simulink model "CryoDetFP"  (R2015b)
settings: Solver=ode45  SolverMode=SingleTasking  StartTime=0.0  StopTime=10e-5  MaxStep=1e-9  RelTol=1e-3
values from neighbouring files (symbols this model uses):
  Fclk = Fadc/2    (= 185000000)    [setupCryoFPGA.m]    (also in setupCryoNew.m)
  freqBusAddrBits = 4    [setupCryoNew.m]
  noise = ifft(exp(2i*pi*rand(1, noiseLen)) .* fft(fir1(noiseLen-1, noiseBW/Fclk*noiseSteps)))    [setupCryoFPGA.m]    (also in setupCryoNew.m = exp(2i*pi*rand(1, noiseLen)))
  noiseLen = 128    [setupCryoFPGA.m]    (also in setupCryoNew.m)
  noiseSteps = 32    [setupCryoFPGA.m]    (also in setupCryoNew.m)
  notch = tf( [1 a*wNotch/Q wNotch^2], [1 wNotch/Q wNotch^2])    [setupCryoNew.m]
  notch2 = tf( [1 a*wNotch/Q wNotch^2], [1 wNotch/Q wNotch^2])    [setupCryoNew.m]
  Tclk = 1/Fclk    (= 5.40540540541e-09)    [setupCryoFPGA.m]    (also in setupCryoNew.m)
undefined symbols (not defined in the file or in its folder): AXI4, Lite, notch3, notch4, xlipgetpartsetting
libraries: xbsIndex_r4 x1085
(part 2 of 8)

== system CryoDetFP/DspCore/AdcDac 0/Ref Delay ==
  note: Delays DAC output data used as Reference for input signal
      | Delay is to compensate for delay of DAC (big), up/downconverter, cable plant, cryostat etc.
      | This is to prevent too much delay mismatch from winding up phase vs. frequency of S21's of sidebands wrt to central line
  In1 : Inport
  Addressable Shift Register : xbsIndex_r4/Addressable Shift Register  infer_latency=on  depth=2  initVector=[0]  en=off  use_behavioral_HDL=on  Optimization=Resource  dbl_ovrd=off  block_type=addrsr
      settings: infoedit="Delay of configurable length.  Any element in the delay line can be addressed and driven onto the output port.<br><br>Hardware notes: Generates fast, compact FIFO-style shift registers or delay lines using SRL16/SRL32 mode of the slice LUTs"
  Addressable Shift Register1 : xbsIndex_r4/Addressable Shift Register  infer_latency=on  depth=2  initVector=[0]  en=off  use_behavioral_HDL=on  Optimization=Resource  dbl_ovrd=off  block_type=addrsr
      settings: infoedit="Delay of configurable length.  Any element in the delay line can be addressed and driven onto the output port.<br><br>Hardware notes: Generates fast, compact FIFO-style shift registers or delay lines using SRL16/SRL32 mode of the slice LUTs"
  Demux : Demux  Outputs=2
  Display : Display
      settings: Decimation=128
  Gateway Out : xbsIndex_r4/Gateway Out  inherit_from_input=off  hdl_port=off  rows=1  columns=1  UseAsDAC=off  DACChannel='1'  interface=None  automatic_assignment=on  address_offset=hex2dec('00')  intf_name=''  intf_description=''  timing_constraint=None  locs_specified=off  LOCs={}  io_standard={}  block_type=gatewayout
  Mux : Mux  Inputs=2
  Out1 : Outport
  wires:
  Addressable Shift Register/1 -> Mux/1
  Addressable Shift Register1/1 -> Mux/2
  In1/1 -> Demux/1
  Demux/2 -> Addressable Shift Register1/1
  Demux/1 -> Addressable Shift Register/1
  [refDel] -> Addressable Shift Register1/2, Addressable Shift Register/2, Gateway Out/1
  Mux/1 -> Out1/1
  Gateway Out/1 -> Display/1

== system CryoDetFP/DspCore/AdcDac 0/SBmodulator ==
  note: To DAC
  note: From tone generators
  note: to sideband demodulators
  note: Band-limited white noise
      | modulator
  note: AM generator
  note: Sideband Modulator
      | Produce sidebands at offset frequency specified by dFsb via amplitude modulation
      | Ampl1 is ratio of sidebands to central line, must be <<1
      | Also provides enable/disable for RF
      | and whitenoise modulator
  In1 : Inport
  AddSub : xbsIndex_r4/AddSub  mode=Addition  use_carryin=off  use_carryout=off  en=off  latency=1  precision=User Defined  arith_type="Signed  (2's comp)"  n_bits=16  bin_pt=15  quantization=Truncate  overflow=Wrap  use_behavioral_HDL=off  hw_selection=Fabric  pipelined=off  dbl_ovrd=off  block_type=addsub
  AddSub1 : xbsIndex_r4/AddSub  mode=Subtraction  use_carryin=off  use_carryout=off  en=off  latency=1  precision=User Defined  arith_type="Signed  (2's comp)"  n_bits=16  bin_pt=15  quantization=Truncate  overflow=Wrap  use_behavioral_HDL=off  hw_selection=Fabric  pipelined=off  dbl_ovrd=off  block_type=addsub
  Concat1 : xbsIndex_r4/Concat  num_inputs=2  dbl_ovrd=off  block_type=concat
  Constant : xbsIndex_r4/Constant  const=1.0  gui_display_data_type=Boolean  arith_type=Boolean  n_bits=16  bin_pt=14  preci_type=Single  exp_width=8  frac_width=24  explicit_period=off  period=1  equ=P=C  opselect=C  inp2=PCIN>>17  opr=+  inp1=P  carry=CIN  dbl_ovrd=off  block_type=constant
  Constant1 : xbsIndex_r4/Constant  const=1.0  gui_display_data_type=Fixed-point  arith_type=Signed (2's comp)  n_bits=16  bin_pt=15  preci_type=Single  exp_width=8  frac_width=24  explicit_period=off  period=1  equ=P=C  opselect=C  inp2=PCIN>>17  opr=+  inp1=P  carry=CIN  dbl_ovrd=off  block_type=constant
  Constant2 : xbsIndex_r4/Constant  const=0  gui_display_data_type=Fixed-point  arith_type=Signed (2's comp)  n_bits=16  bin_pt=15  preci_type=Single  exp_width=8  frac_width=24  explicit_period=off  period=1  equ=P=C  opselect=C  inp2=PCIN>>17  opr=+  inp1=P  carry=CIN  dbl_ovrd=off  block_type=constant
  Counter : xbsIndex_r4/Counter  cnt_type=Free Running  cnt_to=Inf  operation=Up  start_count=0  cnt_by_val=1  arith_type=Unsigned  n_bits=ceil(log2(noiseLen))  bin_pt=0  load_pin=off  rst=off  en=off  explicit_period=on  period=Tclk*noiseSteps  use_behavioral_HDL=off  implementation=Fabric  dbl_ovrd=off  block_type=counter
  "DDS Compiler 6.0 " : xbsIndex_r4/DDS Compiler 6.0   partspresent=Phase_Generator_and_SIN_COS_LUT  dds_clock_rate=Fclk/1e6  channels=1  mode_of_operation=Standard  modulus=9  parameter_entry=Hardware_Parameters  spurious_free_dynamic_range=45  frequency_resolution=0.4  noise_shaping=None  phase_width=16  output_width=16  output_selection=Sine_and_Cosine  negative_sine=off  negative_cosine=off  amplitude_mode=Unit_Circle  memory_type=Auto  optimization_goal=Speed  dsp48_use=Maximal  resync=off  latency_configuration=Auto  latency=5  has_phase_out=off  has_aclken=off  has_aresetn=off  explicit_period=on  period=Tclk  data_has_tlast=Not_Required  has_tready=off  s_phase_has_tuser=Not_Required  m_data_has_tuser=Not_Required  m_phase_has_tuser=Not_Required  s_phase_tuser_width=1  output_form=Twos_Complement  s_config_sync_mode=On_Vector  phase_increment=Programmable  output_frequency1=0  output_frequency2=0  output_frequency3=0  output_frequency4=0  output_frequency5=0  output_frequency6=0  output_frequency7=0  output_frequency8=0  output_frequency9=0  output_frequency10=0  output_frequency11=0  output_frequency12=0  output_frequency13=0  output_frequency14=0  output_frequency15=0  output_frequency16=0  pinc1='0'  pinc2='0'  pinc3='0'  pinc4='0'  pinc5='0'  pinc6='0'  pinc7='0'  pinc8='0'  pinc9='0'  pinc10='0'  pinc11='0'  pinc12='0'  pinc13='0'  pinc14='0'  pinc15='0'  pinc16='0'  phase_offset=None  phase_offset_angles1=0  phase_offset_angles2=0  phase_offset_angles3=0  phase_offset_angles4=0  phase_offset_angles5=0  phase_offset_angles6=0  phase_offset_angles7=0  phase_offset_angles8=0  phase_offset_angles9=0  phase_offset_angles10=0  phase_offset_angles11=0  phase_offset_angles12=0  phase_offset_angles13=0  phase_offset_angles14=0  phase_offset_angles15=0  phase_offset_angles16=0  poff1='0'  poff2='0'  poff3='0'  poff4='0'  poff5='0'  poff6='0'  poff7='0'  poff8='0'  poff9='0'  poff10='0'  poff11='0'  poff12='0'  poff13='0'  poff14='0'  poff15='0'  poff16='0'  trim_axipin_name=on  simulation_type=hybrid_sim  simulation_model=sysgen:xddsv6_0_cmodel  data_path_portlist={ 's_axis_config_tdata_poff', 's_axis_config_tdata_chan0_poff', 's_axis_config_tdata_pinc', 's_axis_config_tdata_chan0_pinc', 's_axis_phase_tdata_resync', 's_axis_phase_tdata_chan0_resync', 's_axis_phase_tdata_poff', 's_axis_phase_tdata_chan0_poff', 's_axis_phase_tdata_pinc', 's_axis_phase_tdata_chan0_pinc', 's_axis_phase_tdata_phase_in', 'm_axis_data_tdata_sine', 'm_axis_data_tdata_chan0_sine', 'm_axis_data_tdata_cosine', 'm_axis_data_tdata_chan0_cosine', 'm_axis_phase_tdata_phase_out', 'm_axis_phase_tdata_chan0_phase_out'}  por_mode=false  gui_behaviour=Sysgen  ip_name=DDS Compiler  ip_version=6.0  dsptool_ready=true  wrapper_available=true  port_translation_map={ 'aclken' => 'en', 'aresetn' => 'rst' }  ipcore_usecache=true  ipcore_useipmodelcache=true  ipcore_xco_need_fpga_part=true  ipcore_fpga_part=xlipgetpartsetting(gcb, {'kintex7', 'xc7k325t', '-3', 'fbg676'})  ipcore_verbose=false  block_type=dds_compiler_v6_0
  Demux : Demux  Outputs=2
  Gateway Out{,1..7} (8 alike) : xbsIndex_r4/Gateway Out  inherit_from_input=off  hdl_port=off  rows=1  columns=1  UseAsDAC=off  DACChannel='1'  interface=None  automatic_assignment=on  address_offset=hex2dec('00')  intf_name=''  intf_description=''  timing_constraint=None  locs_specified=off  LOCs={}  io_standard={}  block_type=gatewayout
  Modulator Control : Display
  Mult : xbsIndex_r4/Mult  precision=User Defined  arith_type="Signed  (2's comp)"  n_bits=16  bin_pt=15  quantization=Truncate  overflow=Wrap  en=off  latency=3  use_behavioral_HDL=off  opt=Speed  use_embedded=on  optimum_pipeline=off  pipeline=on  dbl_ovrd=off  use_rpm=on  placement_style=Triangular  block_type=mult
  Mult1 : xbsIndex_r4/Mult  precision=User Defined  arith_type="Signed  (2's comp)"  n_bits=16  bin_pt=15  quantization=Truncate  overflow=Wrap  en=off  latency=3  use_behavioral_HDL=off  opt=Speed  use_embedded=on  optimum_pipeline=off  pipeline=on  dbl_ovrd=off  use_rpm=on  placement_style=Triangular  block_type=mult
  Mult2 : xbsIndex_r4/Mult  precision=User Defined  arith_type="Signed  (2's comp)"  n_bits=16  bin_pt=15  quantization=Truncate  overflow=Wrap  en=off  latency=3  use_behavioral_HDL=off  opt=Speed  use_embedded=on  optimum_pipeline=off  pipeline=on  dbl_ovrd=off  use_rpm=on  placement_style=Triangular  block_type=mult
  Mux : Mux  Inputs=2
  Mux1 : xbsIndex_r4/Mux  inputs=4  en=off  latency=1  precision=User Defined  arith_type="Signed  (2's comp)"  n_bits=16  bin_pt=15  quantization=Truncate  overflow=Flag as error  dbl_ovrd=off  block_type=mux
  Mux2 : xbsIndex_r4/Mux  inputs=4  en=off  latency=1  precision=User Defined  arith_type="Signed  (2's comp)"  n_bits=16  bin_pt=15  quantization=Truncate  overflow=Flag as error  dbl_ovrd=off  block_type=mux
  Phase Modulator : Subsystem
  ROM : xbsIndex_r4/ROM  depth=noiseLen  initVector=real(noise)  distributed_mem=Block RAM  rst=off  init_reg=0  en=off  latency=1  gui_display_data_type=Fixed-point  arith_type="Signed  (2's comp)"  n_bits=16  bin_pt=15  preci_type=Single  exp_width=8  frac_width=24  optimize=Area  use_rpm=on  dbl_ovrd=off  block_type=sprom
  ROM1 : xbsIndex_r4/ROM  depth=noiseLen  initVector=imag(noise)  distributed_mem=Block RAM  rst=off  init_reg=0  en=off  latency=1  gui_display_data_type=Fixed-point  arith_type="Signed  (2's comp)"  n_bits=16  bin_pt=15  preci_type=Single  exp_width=8  frac_width=24  optimize=Area  use_rpm=on  dbl_ovrd=off  block_type=sprom
  Scope : Scope  NumInputPorts=4
  Terminator : Terminator
  sideband LO : Scope  NumInputPorts=3
  Out1 : Outport
  tag scope: SBI=global, SBQ=global
  wires:
  [dFsb] -> "DDS Compiler 6.0 "/2
  Constant/1 -> "DDS Compiler 6.0 "/1
  Mult/1 -> AddSub/1
  Constant1/1 -> AddSub1/1
  [Ampl1] -> AddSub1/2, Mult/2
  AddSub1/1 -> AddSub/2
  "DDS Compiler 6.0 "/1 -> Terminator/1
  Counter/1 -> ROM1/1, ROM/1
  Demux/1 -> Mult2/1, Phase Modulator/1(Iin)
  Demux/2 -> Phase Modulator/2(Qin), Mult1/1
  Gateway Out/1 -> Scope/1
  Gateway Out1/1 -> Scope/2
  Gateway Out2/1 -> Scope/3
  Gateway Out3/1 -> Scope/4
  "DDS Compiler 6.0 "/3 -> Gateway Out4/1, [SBI], Mult/1
  "DDS Compiler 6.0 "/2 -> Gateway Out5/1, [SBQ]
  Gateway Out4/1 -> sideband LO/1
  Gateway Out5/1 -> sideband LO/2
  [RFen] -> Concat1/2
  Concat1/1 -> Gateway Out6/1, Mux1/1, Mux2/1
  [whiteNoiseGen] -> Concat1/1
  AddSub/1 -> Gateway Out7/1, Mult1/2, Mult2/2
  ROM/1 -> Gateway Out2/1, Phase Modulator/3(Ipm)
  ROM1/1 -> Gateway Out3/1, Phase Modulator/4(Qpm)
  Constant2/1 -> Mux2/4, Mux1/2, Mux1/4, Mux2/2
  Mux2/1 -> Mux/1, Gateway Out/1
  Mux1/1 -> Mux/2, Gateway Out1/1
  Phase Modulator/1(Iout) -> Mux2/5
  Phase Modulator/2(Qout) -> Mux1/5
  Mult2/1 -> Mux2/3
  Mult1/1 -> Mux1/3
  Gateway Out6/1 -> Modulator Control/1
  Gateway Out7/1 -> sideband LO/3
  In1/1 -> Demux/1
  Mux/1 -> Out1/1

== system CryoDetFP/DspCore/AdcDac 0/dF ==
  note: eta Ram has latency 2
  note: sig0
  note: conj(Ref0)
  note: Match latencies
  note: dF
  note: Ref
  note: Sig
  note: Frequency error dF = Im(eta'*Ref'*Sig)
      | where eta' is like a phase and amplitude calibration including the phase determined by the 2 sidebands and amplitude determined by the reference central line and bandwidth
      |
      | get channel ID
      | fetch eta'
      | calc dF
  note: Bandwidth (kludge in with constant for now)
  In1 : Inport
  etaBus : Inport  Port=2
  Bus Creator : BusCreator  Inputs=2
  Bus Selector : BusSelector  OutputSignals=chanAndTvalid,signal2
  CMult : xbsIndex_r4/CMult  const=-1  gui_display_data_type=Floating-point  const_n_bits=24  const_bin_pt=22  float_type=Single  exp_bits=8  fraction_bits=24  en=off  latency=1  precision=Full  arith_type="Signed  (2's comp)"  n_bits=24  bin_pt=22  quantization=Truncate  overflow=Wrap  use_behavioral_HDL=on  mem_type=Distributed RAM  pipeline=off  dbl_ovrd=off  block_type=cmult
  Constant : xbsIndex_r4/Constant  const=0  gui_display_data_type=Fixed-point  arith_type=Unsigned  n_bits=4  bin_pt=0  preci_type=Single  exp_width=8  frac_width=24  explicit_period=off  period=1  equ=P=C  opselect=C  inp2=PCIN>>17  opr=+  inp1=P  carry=CIN  dbl_ovrd=off  block_type=constant
  Constant2 : xbsIndex_r4/Constant  const=1e6/185e6  gui_display_data_type=Floating-point  arith_type=Floating-point  n_bits=16  bin_pt=14  preci_type=Single  exp_width=8  frac_width=24  explicit_period=off  period=1  equ=P=C  opselect=C  inp2=PCIN>>17  opr=+  inp1=P  carry=CIN  dbl_ovrd=off  block_type=constant
  Convert{,1..3} (4 alike) : xbsIndex_r4/Convert  gui_display_data_type=Floating-point  arith_type=Floating-point  n_bits=16  bin_pt=14  float_type=Single  exp_bits=8  fraction_bits=24  quantization=Truncate  overflow=Wrap  en=off  latency=1  pipeline=off  dbl_ovrd=off  block_type=convert
  Convert4 : xbsIndex_r4/Convert  gui_display_data_type=Fixed-point  arith_type="Signed  (2's comp)"  n_bits=32  bin_pt=30  float_type=Single  exp_bits=8  fraction_bits=24  quantization="Round  (unbiased: +/- Inf)"  overflow=Saturate  en=off  latency=1  pipeline=off  dbl_ovrd=off  block_type=convert
  CplxProd : Subsystem
  CplxProd1 : Subsystem
  Delay : xbsIndex_r4/Delay  rst=off  infoeditControl=Selection of Reset will increase slice count due to use of real FFs and instead of SRLs  en=off  latency=1  reg_retiming=on  dbl_ovrd=off  block_type=delay
  Delay1 : xbsIndex_r4/Delay  rst=off  infoeditControl=Selection of Reset will increase slice count due to use of real FFs and instead of SRLs  en=off  latency=1  reg_retiming=on  dbl_ovrd=off  block_type=delay
  Delay2 : xbsIndex_r4/Delay  rst=off  infoeditControl=Selection of Reset will increase slice count due to use of real FFs and instead of SRLs  en=off  latency=1  reg_retiming=on  dbl_ovrd=off  block_type=delay
  Delay3 : xbsIndex_r4/Delay  rst=off  infoeditControl=Selection of Reset will increase slice count due to use of real FFs and instead of SRLs  en=off  latency=18  reg_retiming=on  dbl_ovrd=off  block_type=delay
  Delay4 : xbsIndex_r4/Delay  rst=off  infoeditControl=Selection of Reset will increase slice count due to use of real FFs and instead of SRLs  en=off  latency=6  reg_retiming=on  dbl_ovrd=off  block_type=delay
  Delay5 : xbsIndex_r4/Delay  rst=off  infoeditControl=Selection of Reset will increase slice count due to use of real FFs and instead of SRLs  en=off  latency=2  reg_retiming=on  dbl_ovrd=off  block_type=delay
  Demux : Demux  Outputs=6
  Demux1 : Demux  Outputs=2
  Demux2 : Demux  Outputs=2
  Demux4 : Demux  Outputs=2
  Display2 : Display
  Display3 : Display
  Gateway Out3 : xbsIndex_r4/Gateway Out  inherit_from_input=off  hdl_port=off  rows=1  columns=1  UseAsDAC=off  DACChannel='1'  interface=None  automatic_assignment=on  address_offset=hex2dec('00')  intf_name=''  intf_description=''  timing_constraint=None  locs_specified=off  LOCs={}  io_standard={}  block_type=gatewayout
  Gateway Out4 : xbsIndex_r4/Gateway Out  inherit_from_input=off  hdl_port=off  rows=1  columns=1  UseAsDAC=off  DACChannel='1'  interface=None  automatic_assignment=on  address_offset=hex2dec('00')  intf_name=''  intf_description=''  timing_constraint=None  locs_specified=off  LOCs={}  io_standard={}  block_type=gatewayout
  Mult4 : xbsIndex_r4/Mult  precision=Full  arith_type="Signed  (2's comp)"  n_bits=32  bin_pt=30  quantization="Round  (unbiased: +/- Inf)"  overflow=Saturate  en=off  latency=3  use_behavioral_HDL=off  opt=Speed  use_embedded=on  optimum_pipeline=off  pipeline=on  dbl_ovrd=off  use_rpm=on  placement_style=Triangular  block_type=mult
  Register : xbsIndex_r4/Register  init=0  rst=off  en=on  dbl_ovrd=off  block_type=register
  Relational : xbsIndex_r4/Relational  mode=a=b  op_type=Bool  en=off  latency=0  dbl_ovrd=off  block_type=relational
  Terminator{,2,4..7} (6 alike) : Terminator
  Toolbar : xbsIndex_r4/Toolbar  func=xltoolbar  block_type=toolbar
      settings: infoedit=Toolbar
  dF output : Scope  NumInputPorts=2
  etaRAM : Subsystem
  Out1 : Outport
  wires:
  Demux/1 -> Demux1/1
  Demux/4 -> Demux2/1
  CMult/1 -> CplxProd/4(Im_B)
  Demux2/1 -> Convert2/1
  Demux2/2 -> Convert3/1
  Delay/1 -> CplxProd/5(Re_B)
  Demux1/2 -> Convert1/1
  Demux1/1 -> Convert/1
  Delay1/1 -> CplxProd/2(Im_A)
  CplxProd1/3(Re_Out) -> Terminator/1
  CplxProd1/1(tvalidOut) -> Terminator2/1
  In1/1 -> Bus Selector/1
  Bus Creator/1 -> Out1/1
  Constant2/1 -> Mult4/1
  CplxProd1/2(Im_Out) -> Mult4/2
  Demux/3 -> Terminator5/1
  Demux/2 -> Terminator4/1
  Demux/5 -> Terminator6/1
  Demux/6 -> Terminator7/1
  Demux4/1 -> Delay3/1, Delay4/1
  Demux4/2 -> Delay5/1
  Bus Selector/1 -> Demux4/1  "<chanAndTvalid>"
  Bus Selector/2 -> Demux/1  "<signal2>"
  etaBus/1 -> etaRAM/2("etaBusIn ")
  Delay4/1 -> etaRAM/1(readAddr)
  Mult4/1 -> Convert4/1  "freqError"
  Delay3/1 -> Bus Creator/1, Relational/1, Gateway Out3/1  "channel"
  Convert3/1 -> Delay/1
  Convert2/1 -> CMult/1
  Convert1/1 -> Delay2/1
  Convert/1 -> Delay1/1
  Delay2/1 -> CplxProd/3(Re_A)
  Delay5/1 -> CplxProd/1(tvalidIn)
  CplxProd/2(Im_Out) -> CplxProd1/2(Im_A)
  CplxProd/3(Re_Out) -> CplxProd1/3(Re_A)
  etaRAM/1(etaQ) -> CplxProd1/4(Im_B)
  etaRAM/2(etaI) -> CplxProd1/5(Re_B)
  CplxProd/1(tvalidOut) -> CplxProd1/1(tvalidIn)
  Convert4/1 -> Register/1, Bus Creator/2  "freqError"
  Gateway Out4/1 -> Display3/1, dF output/2
  Gateway Out3/1 -> dF output/1, Display2/1
  Constant/1 -> Relational/2
  Relational/1 -> Register/2
  Register/1 -> Gateway Out4/1

== system CryoDetFP/DspCore/AdcDac 0/dphi ==
  note: check format of Fbus
  note: scale by 1/2 since phase increment per 1/370 = 1/2 of phase increment per 1/185
  note: dPhi
      | calculate complex phase advance for a single sample of ADC input
      | at the frequency of a single channel and send off on dphiBus
  In1 : Inport
  BitBasher : xbsIndex_r4/BitBasher  bitexpr=a={1'b0, b[23:1]}  display_expr=on  sr_1=a  arith_type1=Unsigned  bin_pt1=24  sr_2=2  arith_type2=Unsigned  bin_pt2=0  sr_3=3  arith_type3=Unsigned  bin_pt3=0  sr_4=4  arith_type4=Unsigned  bin_pt4=0  dbl_ovrd=off  block_type=bitbasher
  Bus Creator : BusCreator  Inputs=3
  Constant : xbsIndex_r4/Constant  const=1  gui_display_data_type=Boolean  arith_type=Boolean  n_bits=16  bin_pt=14  preci_type=Single  exp_width=8  frac_width=24  explicit_period=off  period=1  equ=P=C  opselect=C  inp2=PCIN>>17  opr=+  inp1=P  carry=CIN  dbl_ovrd=off  block_type=constant
  Convert : xbsIndex_r4/Convert  gui_display_data_type=Fixed-point  arith_type=Unsigned  n_bits=16  bin_pt=16  float_type=Single  exp_bits=8  fraction_bits=24  quantization="Round  (unbiased: Even Values)"  overflow=Wrap  en=off  latency=1  pipeline=off  dbl_ovrd=off  block_type=convert
  "DDS Compiler 6.0 " : xbsIndex_r4/DDS Compiler 6.0   partspresent=SIN_COS_LUT_only  dds_clock_rate=100  channels=1  mode_of_operation=Standard  modulus=9  parameter_entry=Hardware_Parameters  spurious_free_dynamic_range=45  frequency_resolution=0.4  noise_shaping=None  phase_width=16  output_width=IQbits  output_selection=Sine_and_Cosine  negative_sine=off  negative_cosine=off  amplitude_mode=Unit_Circle  memory_type=Auto  optimization_goal=Speed  dsp48_use=Maximal  resync=off  latency_configuration=Auto  latency=15  has_phase_out=off  has_aclken=off  has_aresetn=off  explicit_period=on  period=Tclk  data_has_tlast=Not_Required  has_tready=off  s_phase_has_tuser=Not_Required  m_data_has_tuser=Not_Required  m_phase_has_tuser=Not_Required  s_phase_tuser_width=1  output_form=Twos_Complement  s_config_sync_mode=On_Vector  phase_increment=Fixed  output_frequency1=0  output_frequency2=0  output_frequency3=0  output_frequency4=0  output_frequency5=0  output_frequency6=0  output_frequency7=0  output_frequency8=0  output_frequency9=0  output_frequency10=0  output_frequency11=0  output_frequency12=0  output_frequency13=0  output_frequency14=0  output_frequency15=0  output_frequency16=0  pinc1='0'  pinc2='0'  pinc3='0'  pinc4='0'  pinc5='0'  pinc6='0'  pinc7='0'  pinc8='0'  pinc9='0'  pinc10='0'  pinc11='0'  pinc12='0'  pinc13='0'  pinc14='0'  pinc15='0'  pinc16='0'  phase_offset=Programmable  phase_offset_angles1=0  phase_offset_angles2=0  phase_offset_angles3=0  phase_offset_angles4=0  phase_offset_angles5=0  phase_offset_angles6=0  phase_offset_angles7=0  phase_offset_angles8=0  phase_offset_angles9=0  phase_offset_angles10=0  phase_offset_angles11=0  phase_offset_angles12=0  phase_offset_angles13=0  phase_offset_angles14=0  phase_offset_angles15=0  phase_offset_angles16=0  poff1='0'  poff2='0'  poff3='0'  poff4='0'  poff5='0'  poff6='0'  poff7='0'  poff8='0'  poff9='0'  poff10='0'  poff11='0'  poff12='0'  poff13='0'  poff14='0'  poff15='0'  poff16='0'  trim_axipin_name=on  simulation_type=hybrid_sim  simulation_model=sysgen:xddsv6_0_cmodel  data_path_portlist={ 's_axis_config_tdata_poff', 's_axis_config_tdata_chan0_poff', 's_axis_config_tdata_pinc', 's_axis_config_tdata_chan0_pinc', 's_axis_phase_tdata_resync', 's_axis_phase_tdata_chan0_resync', 's_axis_phase_tdata_poff', 's_axis_phase_tdata_chan0_poff', 's_axis_phase_tdata_pinc', 's_axis_phase_tdata_chan0_pinc', 's_axis_phase_tdata_phase_in', 'm_axis_data_tdata_sine', 'm_axis_data_tdata_chan0_sine', 'm_axis_data_tdata_cosine', 'm_axis_data_tdata_chan0_cosine', 'm_axis_phase_tdata_phase_out', 'm_axis_phase_tdata_chan0_phase_out'}  por_mode=false  gui_behaviour=Sysgen  ip_name=DDS Compiler  ip_version=6.0  dsptool_ready=true  wrapper_available=true  port_translation_map={ 'aclken' => 'en', 'aresetn' => 'rst' }  ipcore_usecache=true  ipcore_useipmodelcache=true  ipcore_xco_need_fpga_part=true  ipcore_fpga_part=xlipgetpartsetting(gcb, {'kintex7', 'xc7k325t', '-3', 'fbg676'})  ipcore_verbose=false  block_type=dds_compiler_v6_0
  Delay : xbsIndex_r4/Delay  rst=off  infoeditControl=Selection of Reset will increase slice count due to use of real FFs and instead of SRLs  en=off  latency=7  reg_retiming=off  dbl_ovrd=off  block_type=delay
  Display : Display
  Display1 : Display
  Display2 : Display
  Gateway Out{,1..6} (7 alike) : xbsIndex_r4/Gateway Out  inherit_from_input=off  hdl_port=off  rows=1  columns=1  UseAsDAC=off  DACChannel='1'  interface=None  automatic_assignment=on  address_offset=hex2dec('00')  intf_name=''  intf_description=''  timing_constraint=None  locs_specified=off  LOCs={}  io_standard={}  block_type=gatewayout
  Slice : xbsIndex_r4/Slice  nbits=freqBusAddrBits  boolean_output=off  mode=Lower Bit Location + Width  bit1=0  base1=MSB of Input  bit0=freqBits  base0=LSB of Input  dbl_ovrd=off  block_type=slice
  dphi scope : Scope  NumInputPorts=3
  dphi scope1 : Scope  NumInputPorts=3
  Out1 : Outport
  tag scope: dphiBus=scoped
  wires:
  Bus Creator/1 -> [dphiBus], Out1/1
  BitBasher/1 -> Convert/1, Gateway Out4/1
  Delay/1 -> Bus Creator/1, Gateway Out6/1, Gateway Out2/1  "channel"
  Convert/1 -> Gateway Out5/1, "DDS Compiler 6.0 "/2
  Constant/1 -> "DDS Compiler 6.0 "/1
  "DDS Compiler 6.0 "/2 -> Bus Creator/2, Gateway Out/1  "dPhiQ"
  "DDS Compiler 6.0 "/3 -> Bus Creator/3, Gateway Out1/1  "dPhiI"
  Gateway Out/1 -> dphi scope/2, Display/1
  Gateway Out1/1 -> dphi scope/3, Display1/1
  Gateway Out2/1 -> Display2/1
  In1/1 -> BitBasher/1, Slice/1
  Slice/1 -> Gateway Out3/1, Delay/1
  Gateway Out5/1 -> dphi scope1/3
  Gateway Out4/1 -> dphi scope1/2
  Gateway Out3/1 -> dphi scope1/1
  Gateway Out6/1 -> dphi scope/1

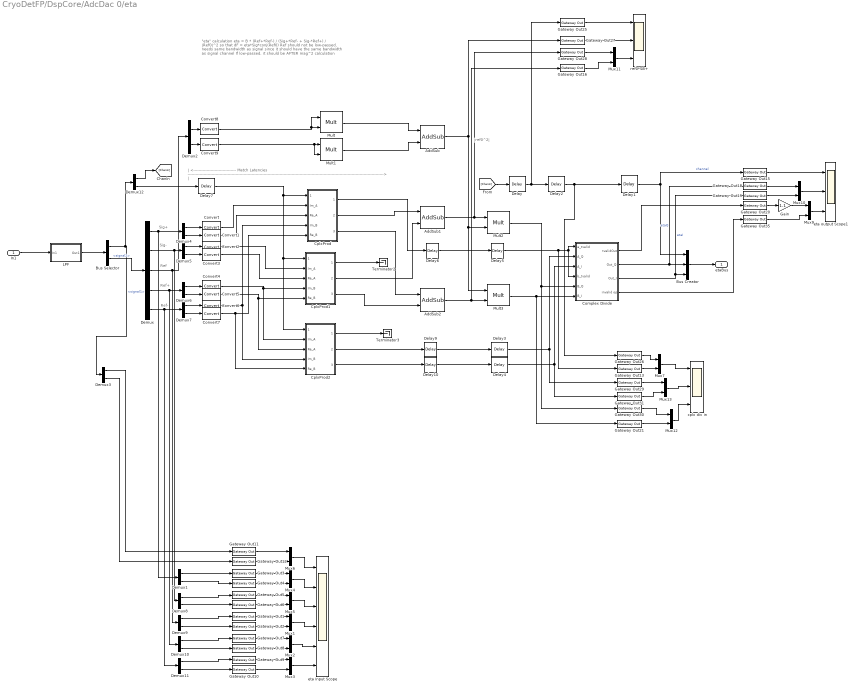
== system CryoDetFP/DspCore/AdcDac 0/eta ==
  note: Sig+
  note: Sig-
  note: Ref+
  note: "eta" calculation
      |
      | eta = B * (Ref+*Ref-) / (Sig+*Ref- + Sig-*Ref+) / |Ref0|^2
      |
      | so that dF = eta*Sig*conj(Ref0)
      |
      | Ref should not be low-passed, needs same bandwidth as signal since it should have the same bandwidth as signal channel
      | If low-passed, it should be AFTER mag^2 calculation
  note: Ref
  note: Ref-
  note: | <-------------------------------- Match Latencies ---------------------------------------------------------------------------------------------------------------------------------------------------> |
  note: |ref0^2|
  In1 : Inport
  AddSub : xbsIndex_r4/AddSub  mode=Addition  use_carryin=off  use_carryout=off  en=off  latency=1  precision=Full  arith_type=Unsigned  n_bits=32  bin_pt=30  quantization="Round  (unbiased: +/- Inf)"  overflow=Saturate  use_behavioral_HDL=off  hw_selection=Fabric  pipelined=off  dbl_ovrd=off  block_type=addsub
  AddSub1 : xbsIndex_r4/AddSub  mode=Addition  use_carryin=off  use_carryout=off  en=off  latency=1  precision=Full  arith_type="Signed  (2's comp)"  n_bits=32  bin_pt=30  quantization="Round  (unbiased: +/- Inf)"  overflow=Saturate  use_behavioral_HDL=off  hw_selection=Fabric  pipelined=off  dbl_ovrd=off  block_type=addsub
  AddSub2 : xbsIndex_r4/AddSub  mode=Addition  use_carryin=off  use_carryout=off  en=off  latency=1  precision=Full  arith_type="Signed  (2's comp)"  n_bits=32  bin_pt=30  quantization="Round  (unbiased: +/- Inf)"  overflow=Saturate  use_behavioral_HDL=off  hw_selection=Fabric  pipelined=off  dbl_ovrd=off  block_type=addsub
  Bus Creator : BusCreator  Inputs=3
  Bus Selector : BusSelector  OutputSignals=signal1,signal2
  Complex Divide : Subsystem
  Convert{,1..9} (10 alike) : xbsIndex_r4/Convert  gui_display_data_type=Floating-point  arith_type=Floating-point  n_bits=16  bin_pt=14  float_type=Single  exp_bits=8  fraction_bits=24  quantization=Truncate  overflow=Wrap  en=off  latency=1  pipeline=off  dbl_ovrd=off  block_type=convert
  CplxProd : Subsystem
  CplxProd1 : Subsystem
  CplxProd2 : Subsystem
  Delay : xbsIndex_r4/Delay  rst=off  infoeditControl=Selection of Reset will increase slice count due to use of real FFs and instead of SRLs  en=off  latency=8  reg_retiming=off  dbl_ovrd=off  block_type=delay
  Delay1 : xbsIndex_r4/Delay  rst=off  infoeditControl=Selection of Reset will increase slice count due to use of real FFs and instead of SRLs  en=off  latency=15  reg_retiming=on  dbl_ovrd=off  block_type=delay
  Delay{6..7,9..10} (4 alike) : xbsIndex_r4/Delay  rst=off  infoeditControl=Selection of Reset will increase slice count due to use of real FFs and instead of SRLs  en=off  latency=1  reg_retiming=off  dbl_ovrd=off  block_type=delay
  Delay{2..5} (4 alike) : xbsIndex_r4/Delay  rst=off  infoeditControl=Selection of Reset will increase slice count due to use of real FFs and instead of SRLs  en=off  latency=3  reg_retiming=off  dbl_ovrd=off  block_type=delay
  Demux : Demux  Outputs=5
  Demux{1..12} (12 alike) : Demux  Outputs=2
  Gain : Gain  Gain=1.1
  Gateway Out{1..13,15..16,18..21,25..31,35} (27 alike) : xbsIndex_r4/Gateway Out  inherit_from_input=off  hdl_port=off  rows=1  columns=1  UseAsDAC=off  DACChannel='1'  interface=None  automatic_assignment=on  address_offset=hex2dec('00')  intf_name=''  intf_description=''  timing_constraint=None  locs_specified=off  LOCs={}  io_standard={}  block_type=gatewayout
  LPF : Subsystem
  Mult : xbsIndex_r4/Mult  precision=Full  arith_type="Signed  (2's comp)"  n_bits=32  bin_pt=30  quantization="Round  (unbiased: +/- Inf)"  overflow=Saturate  en=off  latency=6  use_behavioral_HDL=off  opt=Speed  use_embedded=on  optimum_pipeline=off  pipeline=on  dbl_ovrd=off  use_rpm=on  placement_style=Triangular  block_type=mult
  Mult1 : xbsIndex_r4/Mult  precision=Full  arith_type="Signed  (2's comp)"  n_bits=32  bin_pt=30  quantization="Round  (unbiased: +/- Inf)"  overflow=Saturate  en=off  latency=6  use_behavioral_HDL=off  opt=Speed  use_embedded=on  optimum_pipeline=off  pipeline=on  dbl_ovrd=off  use_rpm=on  placement_style=Triangular  block_type=mult
  Mult2 : xbsIndex_r4/Mult  precision=Full  arith_type="Signed  (2's comp)"  n_bits=32  bin_pt=30  quantization="Round  (unbiased: +/- Inf)"  overflow=Saturate  en=off  latency=3  use_behavioral_HDL=off  opt=Speed  use_embedded=on  optimum_pipeline=off  pipeline=on  dbl_ovrd=off  use_rpm=on  placement_style=Triangular  block_type=mult
  Mult3 : xbsIndex_r4/Mult  precision=Full  arith_type="Signed  (2's comp)"  n_bits=32  bin_pt=30  quantization="Round  (unbiased: +/- Inf)"  overflow=Saturate  en=off  latency=3  use_behavioral_HDL=off  opt=Speed  use_embedded=on  optimum_pipeline=off  pipeline=on  dbl_ovrd=off  use_rpm=on  placement_style=Triangular  block_type=mult
  Mux{1..7,9..13} (12 alike) : Mux  Inputs=2
  Terminator2 : Terminator
  Terminator3 : Terminator
  cplx div in : Scope  NumInputPorts=3
  eta Input Scope : Scope  NumInputPorts=6
  eta output Scope1 : Scope  NumInputPorts=3
  ref0*SB+ : Scope  NumInputPorts=3
  etaBus : Outport
  wires:
  Demux4/1 -> Convert/1
  Demux4/2 -> Convert1/1
  Demux7/1 -> Convert6/1
  Demux7/2 -> Convert7/1
  Demux5/1 -> Convert2/1
  Demux5/2 -> Convert3/1
  Demux6/1 -> Convert4/1
  Demux6/2 -> Convert5/1
  Demux12/2 -> Delay7/1
  AddSub2/1 -> Gateway Out16/1, Mult3/2
  AddSub1/1 -> Gateway Out28/1, Mult2/1
  Mult/1 -> AddSub/1
  Mult1/1 -> AddSub/2
  Demux2/1 -> Convert8/1
  Demux2/2 -> Convert9/1
  CplxProd1/3(Re_Out) -> AddSub2/2
  CplxProd/3(Re_Out) -> AddSub2/1
  CplxProd1/2(Im_Out) -> AddSub1/2
  AddSub/1 -> Mult3/1, Mult2/2, Gateway Out27/1
  Mult2/1 -> Complex Divide/5(B_Q), Gateway Out30/1
  Mult3/1 -> Gateway Out21/1, Complex Divide/6(B_I)
  CplxProd/1(tvalidOut) -> Delay6/1
  CplxProd2/3(Re_Out) -> Delay10/1
  In1/1 -> LPF/1(In1)
  Bus Selector/2 -> Demux/1  "<signal2>"
  [ChanIn] -> Delay/1
  Delay/1 -> Gateway Out25/1, Delay2/1
  LPF/1(Out1) -> Bus Selector/1
  Delay1/1 -> Gateway Out15/1, Bus Creator/1  "channel"
  Complex Divide/2(Out_Q) -> Gateway Out18/1, Bus Creator/2  "etaQ"
  Complex Divide/3(Out_I) -> Gateway Out19/1, Bus Creator/3  "etaI"
  Bus Creator/1 -> etaBus/1
  Bus Selector/1 -> Demux12/1, Demux3/1  "<signal1>"
  Demux3/1 -> Gateway Out11/1
  Demux3/2 -> Gateway Out12/1
  Demux/5 -> Demux11/1, Demux7/1
  Demux/4 -> Demux6/1, Demux10/1
  Demux/2 -> Demux8/1, Demux5/1
  Demux/1 -> Demux4/1, Demux1/1
  Demux/3 -> Demux9/1, Demux2/1
  CplxProd1/1(tvalidOut) -> Terminator2/1
  Gateway Out6/1 -> Mux5/2
  Gateway Out5/1 -> Mux5/1
  Gateway Out4/1 -> Mux4/2
  Gateway Out3/1 -> Mux4/1
  Mux4/1 -> eta Input Scope/2
  Mux5/1 -> eta Input Scope/3
  Gateway Out2/1 -> Mux1/2
  Gateway Out1/1 -> Mux1/1
  Gateway Out8/1 -> Mux2/2
  Gateway Out7/1 -> Mux2/1
  Gateway Out10/1 -> Mux3/2
  Gateway Out9/1 -> Mux3/1
  Mux3/1 -> eta Input Scope/6
  Mux2/1 -> eta Input Scope/5
  Mux1/1 -> eta Input Scope/4
  Demux1/1 -> Gateway Out3/1
  Demux1/2 -> Gateway Out4/1
  Demux8/2 -> Gateway Out6/1
  Demux8/1 -> Gateway Out5/1
  Demux9/2 -> Gateway Out2/1
  Demux9/1 -> Gateway Out1/1
  Demux10/2 -> Gateway Out8/1
  Demux10/1 -> Gateway Out7/1
  Demux11/2 -> Gateway Out10/1
  Demux11/1 -> Gateway Out9/1
  Gateway Out12/1 -> Mux6/2
  Gateway Out11/1 -> Mux6/1
  Mux6/1 -> eta Input Scope/1
  Gateway Out19/1 -> Mux10/2
  Gateway Out18/1 -> Mux10/1
  Mux10/1 -> eta output Scope1/2
  Gateway Out15/1 -> eta output Scope1/1
  Gateway Out25/1 -> ref0*SB+/1
  Gateway Out27/1 -> ref0*SB+/2
  Mux11/1 -> ref0*SB+/3
  Gateway Out28/1 -> Mux11/1
  Gateway Out16/1 -> Mux11/2
  Delay2/1 -> Gateway Out26/1, Delay1/1
  Delay3/1 -> Complex Divide/2(A_Q), Gateway Out29/1
  Delay4/1 -> Complex Divide/3(A_I), Gateway Out31/1
  Mux12/1 -> cplx div in/3
  Gateway Out30/1 -> Mux12/1
  Gateway Out21/1 -> Mux12/2
  Gateway Out29/1 -> Mux13/1
  Mux13/1 -> cplx div in/2
  Gateway Out31/1 -> Mux13/2
  Gateway Out13/1 -> Mux7/2
  Gateway Out26/1 -> Mux7/1
  Mux7/1 -> cplx div in/1
  Demux12/1 -> [ChanIn]
  CplxProd/2(Im_Out) -> AddSub1/1
  Gateway Out20/1 -> Gain/1
  Gateway Out35/1 -> Mux9/2
  Complex Divide/4(invalid op) -> Gateway Out35/1
  Mux9/1 -> eta output Scope1/3
  Gain/1 -> Mux9/1
  Convert/1 -> CplxProd/2(Im_A)
  Convert1/1 -> CplxProd/3(Re_A)
  Convert2/1 -> CplxProd1/2(Im_A)
  Convert3/1 -> CplxProd1/3(Re_A)
  Convert4/1 -> CplxProd2/2(Im_A), CplxProd1/4(Im_B)
  Convert5/1 -> CplxProd2/3(Re_A), CplxProd1/5(Re_B)
  Convert6/1 -> CplxProd2/4(Im_B), CplxProd/4(Im_B)
  Convert7/1 -> CplxProd2/5(Re_B), CplxProd/5(Re_B)
  Convert9/1 -> Mult1/2, Mult1/1
  Convert8/1 -> Mult/1, Mult/2
  Delay6/1 -> Delay5/1
  Delay7/1 -> CplxProd/1(tvalidIn), CplxProd1/1(tvalidIn), CplxProd2/1(tvalidIn)
  CplxProd2/1(tvalidOut) -> Terminator3/1
  Delay10/1 -> Delay4/1
  Delay9/1 -> Delay3/1
  CplxProd2/2(Im_Out) -> Delay9/1
  Delay5/1 -> Gateway Out13/1, Complex Divide/4(b_tvalid), Complex Divide/1(a_tvalid)
  Complex Divide/1(tvalidOut) -> Gateway Out20/1

== system CryoDetFP/DspCore/AdcDac 0/loopFilter ==
  note: convert to MHz
  note: no listener yet
  note: F out should be Fi + DF
      | where DF is integral of frequency error dF subject to limits and FBen
  note: kludge dFbus out for now
      | just stick freq in it for now
  note: loopFilter
      | multi-line feedback block
      | mplement intial frequency, limits, integrator, gain
  In1 : Inport
  Assert : xbsIndex_r4/Assert  assert_type=on  type_source=Explicitly  gui_display_data_type=Fixed-point  arith_type=Unsigned  n_bits=4  bin_pt=0  preci_type=Single  exp_width=8  frac_width=24  assert_rate=on  rate_source=Explicitly  period=Tclk  output_port=on  block_type=assert
  Assert1 : xbsIndex_r4/Assert  assert_type=on  type_source=Explicitly  gui_display_data_type=Fixed-point  arith_type="Signed  (2's comp)"  n_bits=32  bin_pt=30  preci_type=Single  exp_width=8  frac_width=24  assert_rate=on  rate_source=Explicitly  period=Tclk  output_port=on  block_type=assert
  Assert2 : xbsIndex_r4/Assert  assert_type=on  type_source=Explicitly  gui_display_data_type=Boolean  arith_type=Boolean  n_bits=16  bin_pt=14  preci_type=Single  exp_width=8  frac_width=24  assert_rate=on  rate_source=Explicitly  period=Tclk  output_port=on  block_type=assert
  Assert5 : xbsIndex_r4/Assert  assert_type=on  type_source=Explicitly  gui_display_data_type=Fixed-point  arith_type=Unsigned  n_bits=25  bin_pt=0  preci_type=Single  exp_width=8  frac_width=24  assert_rate=on  rate_source=Explicitly  period=Tclk  output_port=on  block_type=assert
  Assert6 : xbsIndex_r4/Assert  assert_type=on  type_source=Explicitly  gui_display_data_type=Fixed-point  arith_type=Unsigned  n_bits=16  bin_pt=16  preci_type=Single  exp_width=8  frac_width=24  assert_rate=on  rate_source=Explicitly  period=Tclk  output_port=on  block_type=assert
  Assert8 : xbsIndex_r4/Assert  assert_type=on  type_source=Explicitly  gui_display_data_type=Fixed-point  arith_type=Unsigned  n_bits=24  bin_pt=24  preci_type=Single  exp_width=8  frac_width=24  assert_rate=on  rate_source=Explicitly  period=Tclk  output_port=on  block_type=assert
  Assert9 : xbsIndex_r4/Assert  assert_type=on  type_source=Explicitly  gui_display_data_type=Fixed-point  arith_type=Unsigned  n_bits=4  bin_pt=0  preci_type=Single  exp_width=8  frac_width=24  assert_rate=on  rate_source=Explicitly  period=Tclk  output_port=on  block_type=assert
  Bus Selector : BusSelector  OutputSignals=channel,freqError
  Concat : xbsIndex_r4/Concat  num_inputs=2  dbl_ovrd=off  block_type=concat
  Constant : xbsIndex_r4/Constant  const=0  gui_display_data_type=Fixed-point  arith_type=Unsigned  n_bits=4  bin_pt=0  preci_type=Single  exp_width=8  frac_width=24  explicit_period=off  period=1  equ=P=C  opselect=C  inp2=PCIN>>17  opr=+  inp1=P  carry=CIN  dbl_ovrd=off  block_type=constant
  Constant1 : xbsIndex_r4/Constant  const=0  gui_display_data_type=Fixed-point  arith_type=Unsigned  n_bits=4  bin_pt=0  preci_type=Single  exp_width=8  frac_width=24  explicit_period=off  period=1  equ=P=C  opselect=C  inp2=PCIN>>17  opr=+  inp1=P  carry=CIN  dbl_ovrd=off  block_type=constant
  Constant2 : xbsIndex_r4/Constant  const=1  gui_display_data_type=Fixed-point  arith_type=Unsigned  n_bits=4  bin_pt=0  preci_type=Single  exp_width=8  frac_width=24  explicit_period=off  period=1  equ=P=C  opselect=C  inp2=PCIN>>17  opr=+  inp1=P  carry=CIN  dbl_ovrd=off  block_type=constant
  Delay2 : xbsIndex_r4/Delay  rst=off  infoeditControl=Selection of Reset will increase slice count due to use of real FFs and instead of SRLs  en=off  latency=3  reg_retiming=off  dbl_ovrd=off  block_type=delay
  Delay3 : xbsIndex_r4/Delay  rst=off  infoeditControl=Selection of Reset will increase slice count due to use of real FFs and instead of SRLs  en=off  latency=3  reg_retiming=off  dbl_ovrd=off  block_type=delay
  Display2 : Display
  Display3 : Display
  Gain1 : Gain  Gain=185
  Gain2 : Gain  Gain=185
  Gain3 : Gain  Gain=185
  Gateway Out12 : xbsIndex_r4/Gateway Out  inherit_from_input=off  hdl_port=off  rows=1  columns=1  UseAsDAC=off  DACChannel='1'  interface=None  automatic_assignment=on  address_offset=hex2dec('00')  intf_name=''  intf_description=''  timing_constraint=None  locs_specified=off  LOCs={}  io_standard={}  block_type=gatewayout
  Gateway Out13 : xbsIndex_r4/Gateway Out  inherit_from_input=on  hdl_port=off  rows=1  columns=1  UseAsDAC=off  DACChannel='1'  interface=None  automatic_assignment=on  address_offset=hex2dec('00')  intf_name=''  intf_description=''  timing_constraint=None  locs_specified=off  LOCs={}  io_standard={}  block_type=gatewayout
  Gateway Out3 : xbsIndex_r4/Gateway Out  inherit_from_input=off  hdl_port=off  rows=1  columns=1  UseAsDAC=off  DACChannel='1'  interface=None  automatic_assignment=on  address_offset=hex2dec('00')  intf_name=''  intf_description=''  timing_constraint=None  locs_specified=off  LOCs={}  io_standard={}  block_type=gatewayout
  Gateway Out4 : xbsIndex_r4/Gateway Out  inherit_from_input=off  hdl_port=off  rows=1  columns=1  UseAsDAC=off  DACChannel='1'  interface=None  automatic_assignment=on  address_offset=hex2dec('00')  intf_name=''  intf_description=''  timing_constraint=None  locs_specified=off  LOCs={}  io_standard={}  block_type=gatewayout
  Gateway Out5 : xbsIndex_r4/Gateway Out  inherit_from_input=on  hdl_port=off  rows=1  columns=1  UseAsDAC=off  DACChannel='1'  interface=None  automatic_assignment=on  address_offset=hex2dec('00')  intf_name=''  intf_description=''  timing_constraint=None  locs_specified=off  LOCs={}  io_standard={}  block_type=gatewayout
  Logical : xbsIndex_r4/Logical  logical_function=OR  inputs=2  en=off  latency=3  precision=User Defined  arith_type=Boolean  n_bits=16  bin_pt=0  align_bp=on  dbl_ovrd=off  block_type=logical
  MCode : xbsIndex_r4/MCode  mfname=multiLineFeedbackpipelined  explicit_period=on  period=Tclk  inputsTable={'boundInpExpr'=>['','','','',''],'inputs'=>['channelNo','deltaF','FBen','Finitial','dFmax']}  outputsTable={'outputs'=>['freq','chanOut'],'suppressOut'=>['off','off']}  enable_stdout=off  enable_debug=off  suppress_output=on  defparams={}  hide_port_list={}  dbl_ovrd=off  block_type=mcode
  Mult : xbsIndex_r4/Mult  precision=User Defined  arith_type="Signed  (2's comp)"  n_bits=32  bin_pt=30  quantization=Truncate  overflow=Saturate  en=off  latency=3  use_behavioral_HDL=off  opt=Speed  use_embedded=on  optimum_pipeline=off  pipeline=on  dbl_ovrd=off  use_rpm=on  placement_style=Triangular  block_type=mult
  Mux : xbsIndex_r4/Mux  inputs=2  en=off  latency=1  precision=Full  arith_type=Unsigned  n_bits=16  bin_pt=14  quantization=Truncate  overflow=Wrap  dbl_ovrd=off  block_type=mux
  Negate : xbsIndex_r4/Negate  precision=Full  arith_type=Unsigned  n_bits=16  bin_pt=14  quantization=Truncate  overflow=Wrap  en=off  latency=1  dbl_ovrd=off  block_type=negate
  Register : xbsIndex_r4/Register  init=0  rst=off  en=on  dbl_ovrd=off  block_type=register
  Register1 : xbsIndex_r4/Register  init=0  rst=off  en=on  dbl_ovrd=off  block_type=register
  Register2 : xbsIndex_r4/Register  init=0  rst=off  en=on  dbl_ovrd=off  block_type=register
  Reinterpret : xbsIndex_r4/Reinterpret  force_arith_type=off  arith_type=Unsigned  force_bin_pt=on  bin_pt=0  block_type=reinterpret
  Relational : xbsIndex_r4/Relational  mode=a=b  op_type=Bool  en=off  latency=0  dbl_ovrd=off  block_type=relational
  Relational1 : xbsIndex_r4/Relational  mode=a=b  op_type=Bool  en=off  latency=0  dbl_ovrd=off  block_type=relational
  Relational2 : xbsIndex_r4/Relational  mode=a=b  op_type=Bool  en=off  latency=0  dbl_ovrd=off  block_type=relational
  Terminator : Terminator
  Terminator1 : Terminator
  initial Frequencies : Subsystem
  loop filter input : Scope  NumInputPorts=2
  loop filter output : Scope  NumInputPorts=3
  Out1 : Outport
  tag scope: dFbus=scoped, freqBus=scoped
  wires:
  In1/1 -> Bus Selector/1
  Bus Selector/1 -> Relational/1, Gateway Out3/1, initial Frequencies/1(channel), Delay3/1  "<channel>"
  Bus Selector/2 -> Mult/1, Register/1  "<freqError>"
  [dFbus] -> Terminator/1
  [FBgain] -> Terminator1/1
  MCode/2 -> Assert9/1, Relational2/2, Gateway Out12/1, Relational1/2  "channel"
  MCode/1 -> Assert8/1, Register2/1, Register1/1  "frequency"
  Concat/1 -> [freqBus], Out1/1, [dFbus]
  [fbPolarity] -> Mux/1
  [FBgain] -> Mux/2, Negate/1
  [FBlimit] -> Assert6/1
  initial Frequencies/1(Fi) -> Delay2/1
  Assert/1 -> MCode/1
  Assert1/1 -> MCode/2
  Assert2/1 -> MCode/3
  Assert5/1 -> MCode/4
  Assert6/1 -> MCode/5
  Assert9/1 -> Concat/1
  Assert8/1 -> Reinterpret/1
  Reinterpret/1 -> Concat/2
  Gateway Out13/1 -> Gain1/1
  Gateway Out12/1 -> loop filter output/1
  Gateway Out4/1 -> Gain2/1
  Gateway Out3/1 -> loop filter input/1, Display2/1
  Constant/1 -> Relational/2
  Relational/1 -> Register/2
  Register/1 -> Gateway Out4/1
  Constant1/1 -> Relational1/1
  Relational1/1 -> Register1/2
  Register1/1 -> Gateway Out13/1
  Gain1/1 -> loop filter output/2
  Gain2/1 -> Display3/1, loop filter input/2
  Constant2/1 -> Relational2/1
  Relational2/1 -> Register2/2
  Register2/1 -> Gateway Out5/1
  Gateway Out5/1 -> Gain3/1
  Gain3/1 -> loop filter output/3
  Negate/1 -> Mux/3
  Mult/1 -> Assert1/1
  Mux/1 -> Mult/2
  [fpgaReset] -> Logical/2
  [FBen] -> Logical/1
  Logical/1 -> Assert2/1
  Delay3/1 -> Assert/1
  Delay2/1 -> Assert5/1
